simulink model "model"  (R2020a)
settings: Solver=FixedStepAuto  StartTime=0.0  StopTime=sim_duration  FixedStep=1/Fs  RelTol=1e-3
values from neighbouring files (symbols this model uses):
  A = 1000    [parametri.m]    (also in resenje_i_parametri.m = 6000)
  DC = 10    [parametri.m]    (also in resenje_i_parametri.m)
  epsilon = 10    [parametri.m]    (also in resenje_i_parametri.m)
  f = 100    [parametri.m]    (also in resenje_i_parametri.m = 50)
  Fs = 2000    [parametri.m]    (also in resenje_i_parametri.m)
libraries: powerlib_meascontrol x4, dspstat3 x2, cstblocks x1, simulink x1
settings Model: Creator=HP  LastModifiedBy=HP
settings DataIOCC: ExternalInput=real_input_tt  LoadExternalInput=on

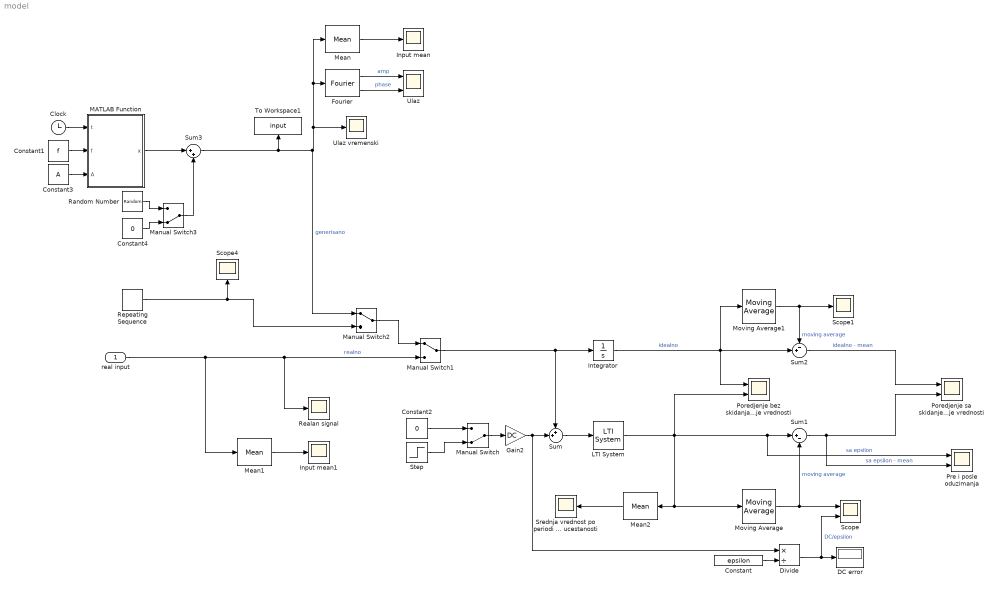
== system model ==
  real input : Inport
  Clock : Clock
  Constant : Constant  Value=epsilon
  Constant1 : Constant  Value=f
  Constant2 : Constant  Value=0
  Constant3 : Constant  Value=A
  Constant4 : Constant  Value=0
  DC error : Display
  Divide : Product  Inputs=*/
  Fourier : powerlib_meascontrol/Measurements/Fourier  Freq=f  n=1  InInit=[0, 0]  Ts=0
  Gain2 : Gain  Gain=DC
  Input mean : Scope
  Input mean1 : Scope
  Integrator : Integrator
  LTI System : cstblocks/LTI System  sys=Gz  IC=[]
  MATLAB Function : MATLAB Function  TreatAsAtomicUnit=on
  Manual Switch : ManualSwitch  CurrentSetting=0
  Manual Switch1 : ManualSwitch
  Manual Switch2 : ManualSwitch
  Manual Switch3 : ManualSwitch  CurrentSetting=0
  Mean : powerlib_meascontrol/Measurements/Mean  Freq=f  Vinit=0  Ts=0
  Mean1 : powerlib_meascontrol/Measurements/Mean  Freq=10  Vinit=0  Ts=0
  Mean2 : powerlib_meascontrol/Measurements/Mean  Freq=40  Vinit=0  Ts=0
  Moving Average : dspstat3/Moving Average  Method=Sliding window  ForgettingFactorPort=off  SpecifyWindowLength=on  WindowLength=2048  ForgettingFactor=0.9  SimulateUsing=Code generation
  Moving Average1 : dspstat3/Moving Average  Method=Sliding window  ForgettingFactorPort=off  SpecifyWindowLength=on  WindowLength=1000  ForgettingFactor=0.9  SimulateUsing=Code generation
  Poredjenje bez skidanja srednje vrednosti : Scope  NumInputPorts=2
  Poredjenje sa skidanjem srednje vrednosti : Scope  NumInputPorts=2
  Pre i posle oduzimanja : Scope  NumInputPorts=2
  Random Number : RandomNumber  Variance=0.01*A  SampleTime=1/Fs
  Realan signal : Scope
  Repeating Sequence : simulink/Sources/Repeating Sequence  rep_seq_t=[0 10 20 30 40] * 1/Fs  rep_seq_y=[0 20 0 -20 0]
  Scope : Scope  NumInputPorts=2
  Scope1 : Scope
  Scope4 : Scope
  Srednja vrednost po periodi neke ucestanosti : Scope
  Step : Step  Time=5  Before=1  After=5  SampleTime=0
  Sum : Sum  Inputs=++|
  Sum1 : Sum  Inputs=|+-
  Sum2 : Sum  Inputs=-+|
  Sum3 : Sum  Inputs=|++
  To Workspace1 : ToWorkspace  VariableName=input  SampleTime=-1
  Ulaz : Scope  NumInputPorts=2
  Ulaz vremenski : Scope
  wires:
  MATLAB Function/1(x) -> Sum3/1
  Sum/1 -> LTI System/1
  LTI System/1 -> Moving Average/1, Mean2/1, Poredjenje bez skidanja srednje vrednosti/2, Pre i posle oduzimanja/1, Sum1/1  "sa epsilon"
  Constant/1 -> Divide/2
  Divide/1 -> Scope/2, DC error/1  "DC/epsilon"
  Fourier/1 -> Ulaz/1  "amp"
  Fourier/2 -> Ulaz/2  "phase"
  Moving Average/1 -> Sum1/2, Scope/1  "moving average"
  Constant1/1 -> MATLAB Function/2(f)
  Gain2/1 -> Divide/1, Sum/2
  Manual Switch/1 -> Gain2/1
  Constant2/1 -> Manual Switch/1
  Step/1 -> Manual Switch/2
  Mean/1 -> Input mean/1
  Clock/1 -> MATLAB Function/1(t)
  Constant3/1 -> MATLAB Function/3(A)
  Integrator/1 -> Moving Average1/1, Sum2/2, Poredjenje bez skidanja srednje vrednosti/1  "idealno"
  Sum1/1 -> Pre i posle oduzimanja/2, Poredjenje sa skidanjem srednje vrednosti/2  "sa epsilon - mean"
  Moving Average1/1 -> Scope1/1, Sum2/1  "moving average"
  Sum2/1 -> Poredjenje sa skidanjem srednje vrednosti/1  "idealno - mean"
  Sum3/1 -> Manual Switch2/1, Mean/1, Fourier/1, Ulaz vremenski/1, To Workspace1/1  "generisano"
  real input/1 -> Mean1/1, Realan signal/1, Manual Switch1/2  "realno"
  Mean1/1 -> Input mean1/1
  Manual Switch1/1 -> Sum/1, Integrator/1
  Mean2/1 -> Srednja vrednost po periodi neke ucestanosti/1
  Manual Switch2/1 -> Manual Switch1/1
  Repeating Sequence/1 -> Manual Switch2/2, Scope4/1
  Random Number/1 -> Manual Switch3/1
  Constant4/1 -> Manual Switch3/2
  Manual Switch3/1 -> Sum3/2

== matlab function model/MATLAB Function ==
  data: t input; x output; f input; A input
function x = input_signal(t, f, A)
    x = 0;
    n = 1;
    for i = 1:n
        x = x + A/i * cos(2*pi* i*f * t + pi/6 * i);
    end
end
